simulink model "Q2"  (R2022b)
settings: Solver=FixedStepAuto  StartTime=0.0  StopTime=10.0  FixedStep=1  RelTol=1e-3
undefined symbols (not defined in the file): sigbuilder_block
settings Model: Creator=Erfan  LastModifiedBy=Erfan

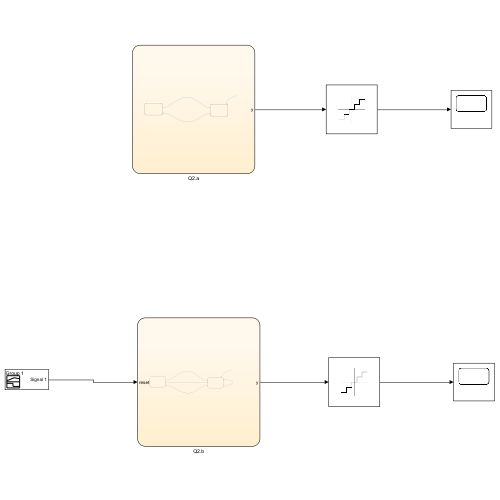
[thumbnail: Simulink's stored preview of the top-level diagram]
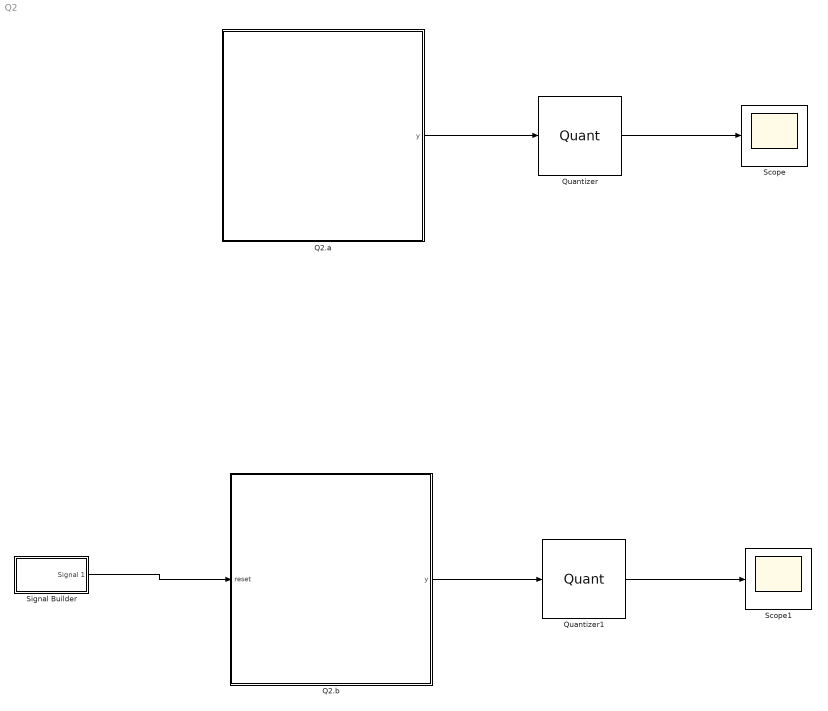
== system Q2 ==
  Q2.a : Stateflow chart  TreatAsAtomicUnit=on
  Q2.b : Stateflow chart  TreatAsAtomicUnit=on
  Quantizer : Quantizer
  Quantizer1 : Quantizer
  Scope : Scope
  Scope1 : Scope
  Signal Builder : Subsystem  Tag=STV Subsys  LoadFcn=sigbuilder_block('load',[437.6 199.2 550.4 400 ]);  StartFcn=sigbuilder_block('start');  StopFcn=sigbuilder_block('stop');  ClipboardFcn=sigbuilder_block('clipboard');  mask(Sigbuilder block){tuvar=[0:10]}
      mask help: Simulink:masks:SigbuilderBlock_MD
      mask init:
      | if ~strcmp(get_param(bdroot(gcbh),'SimulationStatus'),'stopped') tuvar = sigbuilder_block('maskInit'); end
      settings: CopyFcn=sigbuilder_block('copy');  DeleteFcn=sigbuilder_block('delete');  ModelCloseFcn=sigbuilder_block('modelClose');  PreSaveFcn=sigbuilder_block('preSave');  PauseFcn=sigbuilder_block('pause');  ContinueFcn=sigbuilder_block('continue');  NameChangeFcn=sigbuilder_block('namechange');  OpenFcn=sigbuilder_block('open',[437.6 199.2 550.4 400 ]);  CloseFcn=sigbuilder_block('close');
      mask Display: plot(0, 0, 100, 100,[2, 2, 32, 32, 2], [68, 8, 8, 68, 68],[32, 2], [38, 38], [32, 19, 2],[53, 60, 44], [32, 17, 17, 2],[16, 16, 31, 31]);txt = getActiveGroup(gcbh);text(2, 100, txt,'verticalAlignment', 'top');
  wires:
  Q2.a/1(y) -> Quantizer/1
  Quantizer/1 -> Scope/1
  Q2.b/1(y) -> Quantizer1/1
  Quantizer1/1 -> Scope1/1
  Signal Builder/1(Signal 1) -> Q2.b/1(reset)

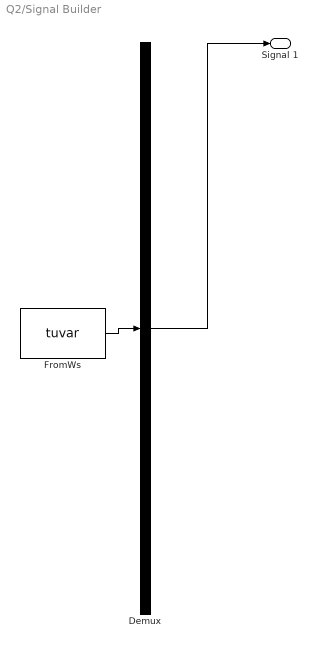
== system Q2/Signal Builder ==
  Demux : Demux  Tag=STV Demux  Outputs=1
      settings: DisplayOption=none
  FromWs : FromWorkspace  Tag=STV FromWs  VariableName=tuvar
      SigBuilderData=|
      | common.afterFinalStr = 'Extrapolate'
      | common.sampleTime = 0
      | dataSet.timeRange = [0 10]
      | dataSet.name = 'Group 1'
      | sbobj.Groups.Name = 'Group 1'
      | sbobj.Groups.Signals.Name = 'Signal 1'
      | sbobj.Groups.Signals.XData = [0 2 2 6 6 10]
      | sbobj.Groups.Signals.YData = [0 0 1 1 0 0]
  Signal 1 : Outport  Tag=STV Outport
  wires:
  Demux/1 -> Signal 1/1
  FromWs/1 -> Demux/1

== stateflow chart Q2/Q2.b ==
  settings: updateMethod=CONTINUOUS
  state Two
    during :
    s_dot = 1;
    r_dot = 1;
  state One
    during:
    s_dot = 1;
    r_dot = 1;
  (default) -> One : {r=0;
      | s=0;}
  Two -> One [order 1] : [r == 2 && reset == 0 ] {y = s; r = 0;}
  One -> One [order 2] : [reset == 1]{s = 0; r = 0;}
  Two -> One [order 2] : [reset == 1]{s = 0; r = 0;}
  One -> Two [order 1] : [r == 1 && reset == 0] {y = s; r = 0; }
  data: r local; s local; y output; reset input
  data r settings: updateMethod=SF_CONTINUOUS_TIME_DATA
  data s settings: updateMethod=SF_CONTINUOUS_TIME_DATA

== stateflow chart Q2/Q2.a ==
  settings: updateMethod=CONTINUOUS
  state Two
    during :
    s_dot = 1;
    r_dot = 1;
  state One
    during:
    s_dot = 1;
    r_dot = 1;
  (default) -> One : {r=0;
      | s=0;}
  Two -> One : [r == 2] {y = s; r = 0;}
  One -> Two : [r == 1] {y = s; r = 0; }
  data: r local; s local; y output
  data r settings: updateMethod=SF_CONTINUOUS_TIME_DATA
  data s settings: updateMethod=SF_CONTINUOUS_TIME_DATA
